simulink model "fusionAlg"  (R2018b)
settings: Solver=FixedStepDiscrete  StartTime=0.0  StopTime=inf  FixedStep=0.01  RelTol=1e-3
PostLoadFcn:
  | if any(exist('dsrtsu_mdlpostloadfcn', 'file') ~= 0), dsrtsu_mdlpostloadfcn('Execute', bdroot); end
model workspace (MAT data in the model file):
  handle : class17 (value not decoded)
(part 4 of 24)

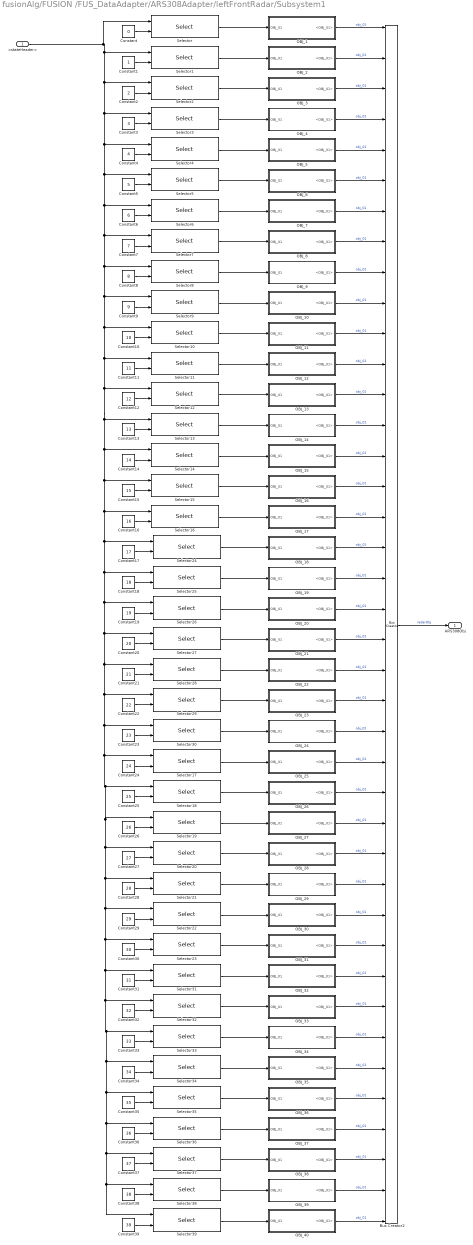
== system fusionAlg/FUSION /FUS_DataAdapter/ARS308Adapter/leftFrontRadar/Subsystem1 ==
  <stateHeader> : Inport
  Bus Creator2 : BusCreator  Inputs=40  OutDataTypeStr=Bus: FUS_RADOBJ_LIST_ST  NonVirtualBus=on
      settings: InheritFromInputs=off
  Constant : Constant  Value=0  OutDataTypeStr=uint8
  Constant1 : Constant  OutDataTypeStr=uint8
  Constant10 : Constant  Value=10  OutDataTypeStr=uint8
  Constant11 : Constant  Value=11  OutDataTypeStr=uint8
  Constant12 : Constant  Value=12  OutDataTypeStr=uint8
  Constant13 : Constant  Value=13  OutDataTypeStr=uint8
  Constant14 : Constant  Value=14  OutDataTypeStr=uint8
  Constant15 : Constant  Value=15  OutDataTypeStr=uint8
  Constant16 : Constant  Value=16  OutDataTypeStr=uint8
  Constant17 : Constant  Value=17  OutDataTypeStr=uint8
  Constant18 : Constant  Value=18  OutDataTypeStr=uint8
  Constant19 : Constant  Value=19  OutDataTypeStr=uint8
  Constant2 : Constant  Value=2  OutDataTypeStr=uint8
  Constant20 : Constant  Value=20  OutDataTypeStr=uint8
  Constant21 : Constant  Value=21  OutDataTypeStr=uint8
  Constant22 : Constant  Value=22  OutDataTypeStr=uint8
  Constant23 : Constant  Value=23  OutDataTypeStr=uint8
  Constant24 : Constant  Value=24  OutDataTypeStr=uint8
  Constant25 : Constant  Value=25  OutDataTypeStr=uint8
  Constant26 : Constant  Value=26  OutDataTypeStr=uint8
  Constant27 : Constant  Value=27  OutDataTypeStr=uint8
  Constant28 : Constant  Value=28  OutDataTypeStr=uint8
  Constant29 : Constant  Value=29  OutDataTypeStr=uint8
  Constant3 : Constant  Value=3  OutDataTypeStr=uint8
  Constant30 : Constant  Value=30  OutDataTypeStr=uint8
  Constant31 : Constant  Value=31  OutDataTypeStr=uint8
  Constant32 : Constant  Value=32  OutDataTypeStr=uint8
  Constant33 : Constant  Value=33  OutDataTypeStr=uint8
  Constant34 : Constant  Value=34  OutDataTypeStr=uint8
  Constant35 : Constant  Value=35  OutDataTypeStr=uint8
  Constant36 : Constant  Value=36  OutDataTypeStr=uint8
  Constant37 : Constant  Value=37  OutDataTypeStr=uint8
  Constant38 : Constant  Value=38  OutDataTypeStr=uint8
  Constant39 : Constant  Value=39  OutDataTypeStr=uint8
  Constant4 : Constant  Value=4  OutDataTypeStr=uint8
  Constant5 : Constant  Value=5  OutDataTypeStr=uint8
  Constant6 : Constant  Value=6  OutDataTypeStr=uint8
  Constant7 : Constant  Value=7  OutDataTypeStr=uint8
  Constant8 : Constant  Value=8  OutDataTypeStr=uint8
  Constant9 : Constant  Value=9  OutDataTypeStr=uint8
  OBJ_1 : Subsystem
  OBJ_10 : Subsystem
  OBJ_11 : Subsystem
  OBJ_12 : Subsystem
  OBJ_13 : Subsystem
  OBJ_14 : Subsystem
  OBJ_15 : Subsystem
  OBJ_16 : Subsystem
  OBJ_17 : Subsystem
  OBJ_18 : Subsystem
  OBJ_19 : Subsystem
  OBJ_2 : Subsystem
  OBJ_20 : Subsystem
  OBJ_21 : Subsystem
  OBJ_22 : Subsystem
  OBJ_23 : Subsystem
  OBJ_24 : Subsystem
  OBJ_25 : Subsystem
  OBJ_26 : Subsystem
  OBJ_27 : Subsystem
  OBJ_28 : Subsystem
  OBJ_29 : Subsystem
  OBJ_3 : Subsystem
  OBJ_30 : Subsystem
  OBJ_31 : Subsystem
  OBJ_32 : Subsystem
  OBJ_33 : Subsystem
  OBJ_34 : Subsystem
  OBJ_35 : Subsystem
  OBJ_36 : Subsystem
  OBJ_37 : Subsystem
  OBJ_38 : Subsystem
  OBJ_39 : Subsystem
  OBJ_4 : Subsystem
  OBJ_40 : Subsystem
  OBJ_5 : Subsystem
  OBJ_6 : Subsystem
  OBJ_7 : Subsystem
  OBJ_8 : Subsystem
  OBJ_9 : Subsystem
  Selector{,1..39} (40 alike) : Selector  IndexMode=Zero-based  InputPortWidth=40  IndexOptions=Index vector (port)  Indices=[1 3]  OutputSizes=1
  ARS308Obj : Outport
  wires:
  Bus Creator2/1 -> ARS308Obj/1  "radarObj"
  Constant/1 -> Selector/2
  Constant11/1 -> Selector11/2
  Constant2/1 -> Selector2/2
  Constant5/1 -> Selector5/2
  Constant26/1 -> Selector19/2
  Constant3/1 -> Selector3/2
  Constant34/1 -> Selector34/2
  Constant22/1 -> Selector29/2
  Constant9/1 -> Selector9/2
  Constant38/1 -> Selector38/2
  Constant14/1 -> Selector14/2
  Constant23/1 -> Selector30/2
  Constant1/1 -> Selector1/2
  Constant6/1 -> Selector6/2
  Constant4/1 -> Selector4/2
  Constant8/1 -> Selector8/2
  <stateHeader>/1 -> Selector/1, Selector9/1, Selector39/1, Selector38/1, Selector37/1, Selector36/1, Selector35/1, Selector34/1, Selector33/1, Selector32/1, Selector31/1, Selector23/1, Selector22/1, Selector21/1, Selector20/1, Selector19/1, Selector18/1, Selector17/1, Selector30/1, Selector29/1, Selector28/1, Selector27/1, Selector26/1, Selector25/1, Selector24/1, Selector16/1, Selector15/1, Selector14/1, Selector13/1, Selector12/1, Selector11/1, Selector10/1, Selector8/1, Selector7/1, Selector6/1, Selector5/1, Selector4/1, Selector3/1, Selector2/1, Selector1/1
  Selector/1 -> OBJ_1/1(OBJ_01)
  Constant17/1 -> Selector24/2
  Constant12/1 -> Selector12/2
  Constant20/1 -> Selector27/2
  Constant39/1 -> Selector39/2
  Constant37/1 -> Selector37/2
  Constant36/1 -> Selector36/2
  Constant15/1 -> Selector15/2
  Constant10/1 -> Selector10/2
  Constant18/1 -> Selector25/2
  Constant19/1 -> Selector26/2
  Constant16/1 -> Selector16/2
  Constant25/1 -> Selector18/2
  Constant28/1 -> Selector21/2
  Constant31/1 -> Selector31/2
  Constant29/1 -> Selector22/2
  Constant13/1 -> Selector13/2
  Constant33/1 -> Selector33/2
  Constant32/1 -> Selector32/2
  Constant24/1 -> Selector17/2
  Constant21/1 -> Selector28/2
  Constant30/1 -> Selector23/2
  Constant27/1 -> Selector20/2
  Constant7/1 -> Selector7/2
  Constant35/1 -> Selector35/2
  OBJ_1/1(<OBJ_01>) -> Bus Creator2/1  "obj_01"
  Selector1/1 -> OBJ_2/1(OBJ_01)
  OBJ_2/1(<OBJ_01>) -> Bus Creator2/2  "obj_01"
  Selector2/1 -> OBJ_3/1(OBJ_01)
  Selector3/1 -> OBJ_4/1(OBJ_01)
  OBJ_4/1(<OBJ_01>) -> Bus Creator2/4  "obj_01"
  OBJ_3/1(<OBJ_01>) -> Bus Creator2/3  "obj_01"
  Selector7/1 -> OBJ_8/1(OBJ_01)
  Selector4/1 -> OBJ_5/1(OBJ_01)
  Selector5/1 -> OBJ_6/1(OBJ_01)
  Selector6/1 -> OBJ_7/1(OBJ_01)
  OBJ_7/1(<OBJ_01>) -> Bus Creator2/7  "obj_01"
  OBJ_6/1(<OBJ_01>) -> Bus Creator2/6  "obj_01"
  OBJ_5/1(<OBJ_01>) -> Bus Creator2/5  "obj_01"
  OBJ_8/1(<OBJ_01>) -> Bus Creator2/8  "obj_01"
  Selector8/1 -> OBJ_9/1(OBJ_01)
  Selector10/1 -> OBJ_11/1(OBJ_01)
  OBJ_10/1(<OBJ_01>) -> Bus Creator2/10  "obj_01"
  OBJ_11/1(<OBJ_01>) -> Bus Creator2/11  "obj_01"
  Selector12/1 -> OBJ_13/1(OBJ_01)
  Selector9/1 -> OBJ_10/1(OBJ_01)
  Selector11/1 -> OBJ_12/1(OBJ_01)
  OBJ_9/1(<OBJ_01>) -> Bus Creator2/9  "obj_01"
  OBJ_13/1(<OBJ_01>) -> Bus Creator2/13  "obj_01"
  OBJ_12/1(<OBJ_01>) -> Bus Creator2/12  "obj_01"
  Selector13/1 -> OBJ_14/1(OBJ_01)
  OBJ_17/1(<OBJ_01>) -> Bus Creator2/17  "obj_01"
  OBJ_14/1(<OBJ_01>) -> Bus Creator2/14  "obj_01"
  OBJ_16/1(<OBJ_01>) -> Bus Creator2/16  "obj_01"
  OBJ_15/1(<OBJ_01>) -> Bus Creator2/15  "obj_01"
  Selector15/1 -> OBJ_16/1(OBJ_01)
  Selector14/1 -> OBJ_15/1(OBJ_01)
  Selector16/1 -> OBJ_17/1(OBJ_01)
  Selector27/1 -> OBJ_21/1(OBJ_01)
  Selector26/1 -> OBJ_20/1(OBJ_01)
  OBJ_18/1(<OBJ_01>) -> Bus Creator2/18  "obj_01"
  OBJ_20/1(<OBJ_01>) -> Bus Creator2/20  "obj_01"
  OBJ_19/1(<OBJ_01>) -> Bus Creator2/19  "obj_01"
  Selector24/1 -> OBJ_18/1(OBJ_01)
  OBJ_21/1(<OBJ_01>) -> Bus Creator2/21  "obj_01"
  Selector25/1 -> OBJ_19/1(OBJ_01)
  Selector28/1 -> OBJ_22/1(OBJ_01)
  OBJ_22/1(<OBJ_01>) -> Bus Creator2/22  "obj_01"
  Selector17/1 -> OBJ_25/1(OBJ_01)
  Selector30/1 -> OBJ_24/1(OBJ_01)
  Selector29/1 -> OBJ_23/1(OBJ_01)
  OBJ_24/1(<OBJ_01>) -> Bus Creator2/24  "obj_01"
  OBJ_23/1(<OBJ_01>) -> Bus Creator2/23  "obj_01"
  OBJ_25/1(<OBJ_01>) -> Bus Creator2/25  "obj_01"
  OBJ_26/1(<OBJ_01>) -> Bus Creator2/26  "obj_01"
  Selector18/1 -> OBJ_26/1(OBJ_01)
  Selector22/1 -> OBJ_30/1(OBJ_01)
  OBJ_27/1(<OBJ_01>) -> Bus Creator2/27  "obj_01"
  Selector21/1 -> OBJ_29/1(OBJ_01)
  OBJ_30/1(<OBJ_01>) -> Bus Creator2/30  "obj_01"
  Selector20/1 -> OBJ_28/1(OBJ_01)
  Selector19/1 -> OBJ_27/1(OBJ_01)
  Selector23/1 -> OBJ_31/1(OBJ_01)
  OBJ_31/1(<OBJ_01>) -> Bus Creator2/31  "obj_01"
  OBJ_29/1(<OBJ_01>) -> Bus Creator2/29  "obj_01"
  OBJ_28/1(<OBJ_01>) -> Bus Creator2/28  "obj_01"
  OBJ_33/1(<OBJ_01>) -> Bus Creator2/33  "obj_01"
  OBJ_34/1(<OBJ_01>) -> Bus Creator2/34  "obj_01"
  Selector34/1 -> OBJ_35/1(OBJ_01)
  Selector33/1 -> OBJ_34/1(OBJ_01)
  Selector32/1 -> OBJ_33/1(OBJ_01)
  OBJ_32/1(<OBJ_01>) -> Bus Creator2/32  "obj_01"
  OBJ_36/1(<OBJ_01>) -> Bus Creator2/36  "obj_01"
  Selector35/1 -> OBJ_36/1(OBJ_01)
  OBJ_35/1(<OBJ_01>) -> Bus Creator2/35  "obj_01"
  Selector31/1 -> OBJ_32/1(OBJ_01)
  Selector39/1 -> OBJ_40/1(OBJ_01)
  OBJ_37/1(<OBJ_01>) -> Bus Creator2/37  "obj_01"
  Selector36/1 -> OBJ_37/1(OBJ_01)
  Selector38/1 -> OBJ_39/1(OBJ_01)
  OBJ_38/1(<OBJ_01>) -> Bus Creator2/38  "obj_01"
  OBJ_40/1(<OBJ_01>) -> Bus Creator2/40  "obj_01"
  Selector37/1 -> OBJ_38/1(OBJ_01)
  OBJ_39/1(<OBJ_01>) -> Bus Creator2/39  "obj_01"

== system fusionAlg/FUSION /FUS_DataAdapter/ARS308Adapter/leftFrontRadar/Subsystem40 ==
  <MeasCounter> : Inport
  Bus Creator1 : BusCreator  Inputs=12  OutDataTypeStr=Bus: FUS_RADAR_STATE_ST  NonVirtualBus=on
      settings: InheritFromInputs=off
  Bus Creator2 : BusCreator  Inputs=2  OutDataTypeStr=Bus: FUS_UINT8_RESERVED_ST  NonVirtualBus=on
      settings: InheritFromInputs=off
  Constant{,1,5..11} (9 alike) : Constant  Value=0  OutDataTypeStr=uint8
  Constant2 : Constant  Value=0  OutDataTypeStr=single
  Constant3 : Constant  Value=0  OutDataTypeStr=single
  Constant4 : Constant  Value=0  OutDataTypeStr=uint16
  Data Type Conversion : DataTypeConversion  OutDataTypeStr=uint8
  <STATUS> : Outport
  wires:
  Constant/1 -> Bus Creator2/1
  <MeasCounter>/1 -> Data Type Conversion/1
  Constant1/1 -> Bus Creator2/2
  Bus Creator2/1 -> Bus Creator1/12
  Bus Creator1/1 -> <STATUS>/1
  Constant2/1 -> Bus Creator1/1  "hostYaw"
  Constant3/1 -> Bus Creator1/2  "hostSpeed"
  Constant4/1 -> Bus Creator1/3  "timestamp"
  Constant5/1 -> Bus Creator1/4  "HWError"
  Constant6/1 -> Bus Creator1/5  "BlkProg"
  Constant7/1 -> Bus Creator1/6  "MisAlign"
  Constant8/1 -> Bus Creator1/7  "GUFail"
  Constant9/1 -> Bus Creator1/8  "measEnabled"
  Constant10/1 -> Bus Creator1/10  "latency"
  Constant11/1 -> Bus Creator1/11  "msgCheckSum"
  Data Type Conversion/1 -> Bus Creator1/9

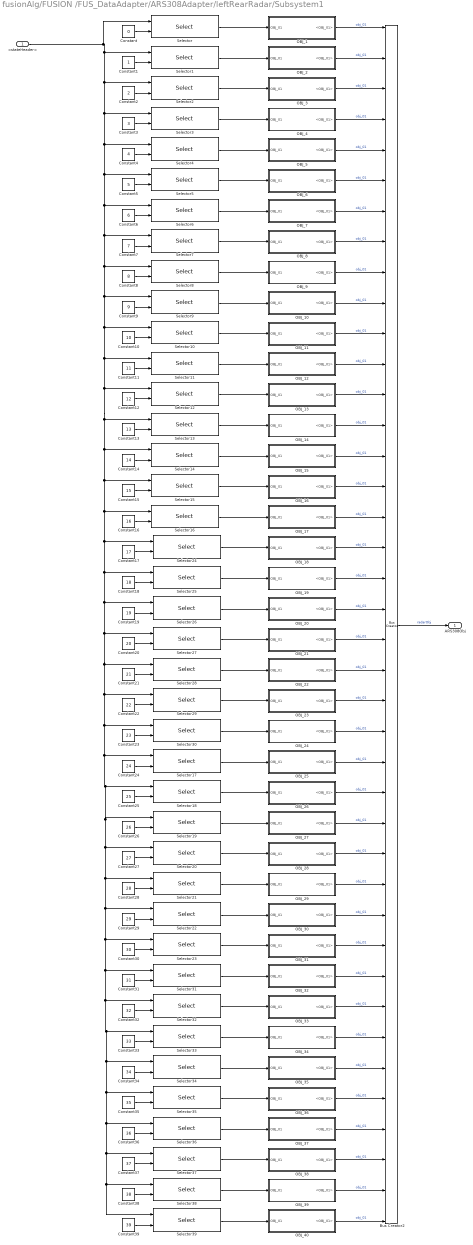
== system fusionAlg/FUSION /FUS_DataAdapter/ARS308Adapter/leftRearRadar/Subsystem1 ==
  <stateHeader> : Inport
  Bus Creator2 : BusCreator  Inputs=40  OutDataTypeStr=Bus: FUS_RADOBJ_LIST_ST  NonVirtualBus=on
      settings: InheritFromInputs=off
  Constant : Constant  Value=0  OutDataTypeStr=uint8
  Constant1 : Constant  OutDataTypeStr=uint8
  Constant10 : Constant  Value=10  OutDataTypeStr=uint8
  Constant11 : Constant  Value=11  OutDataTypeStr=uint8
  Constant12 : Constant  Value=12  OutDataTypeStr=uint8
  Constant13 : Constant  Value=13  OutDataTypeStr=uint8
  Constant14 : Constant  Value=14  OutDataTypeStr=uint8
  Constant15 : Constant  Value=15  OutDataTypeStr=uint8
  Constant16 : Constant  Value=16  OutDataTypeStr=uint8
  Constant17 : Constant  Value=17  OutDataTypeStr=uint8
  Constant18 : Constant  Value=18  OutDataTypeStr=uint8
  Constant19 : Constant  Value=19  OutDataTypeStr=uint8
  Constant2 : Constant  Value=2  OutDataTypeStr=uint8
  Constant20 : Constant  Value=20  OutDataTypeStr=uint8
  Constant21 : Constant  Value=21  OutDataTypeStr=uint8
  Constant22 : Constant  Value=22  OutDataTypeStr=uint8
  Constant23 : Constant  Value=23  OutDataTypeStr=uint8
  Constant24 : Constant  Value=24  OutDataTypeStr=uint8
  Constant25 : Constant  Value=25  OutDataTypeStr=uint8
  Constant26 : Constant  Value=26  OutDataTypeStr=uint8
  Constant27 : Constant  Value=27  OutDataTypeStr=uint8
  Constant28 : Constant  Value=28  OutDataTypeStr=uint8
  Constant29 : Constant  Value=29  OutDataTypeStr=uint8
  Constant3 : Constant  Value=3  OutDataTypeStr=uint8
  Constant30 : Constant  Value=30  OutDataTypeStr=uint8
  Constant31 : Constant  Value=31  OutDataTypeStr=uint8
  Constant32 : Constant  Value=32  OutDataTypeStr=uint8
  Constant33 : Constant  Value=33  OutDataTypeStr=uint8
  Constant34 : Constant  Value=34  OutDataTypeStr=uint8
  Constant35 : Constant  Value=35  OutDataTypeStr=uint8
  Constant36 : Constant  Value=36  OutDataTypeStr=uint8
  Constant37 : Constant  Value=37  OutDataTypeStr=uint8
  Constant38 : Constant  Value=38  OutDataTypeStr=uint8
  Constant39 : Constant  Value=39  OutDataTypeStr=uint8
  Constant4 : Constant  Value=4  OutDataTypeStr=uint8
  Constant5 : Constant  Value=5  OutDataTypeStr=uint8
  Constant6 : Constant  Value=6  OutDataTypeStr=uint8
  Constant7 : Constant  Value=7  OutDataTypeStr=uint8
  Constant8 : Constant  Value=8  OutDataTypeStr=uint8
  Constant9 : Constant  Value=9  OutDataTypeStr=uint8
  OBJ_1 : Subsystem
  OBJ_10 : Subsystem
  OBJ_11 : Subsystem
  OBJ_12 : Subsystem
  OBJ_13 : Subsystem
  OBJ_14 : Subsystem
  OBJ_15 : Subsystem
  OBJ_16 : Subsystem
  OBJ_17 : Subsystem
  OBJ_18 : Subsystem
  OBJ_19 : Subsystem
  OBJ_2 : Subsystem
  OBJ_20 : Subsystem
  OBJ_21 : Subsystem
  OBJ_22 : Subsystem
  OBJ_23 : Subsystem
  OBJ_24 : Subsystem
  OBJ_25 : Subsystem
  OBJ_26 : Subsystem
  OBJ_27 : Subsystem
  OBJ_28 : Subsystem
  OBJ_29 : Subsystem
  OBJ_3 : Subsystem
  OBJ_30 : Subsystem
  OBJ_31 : Subsystem
  OBJ_32 : Subsystem
  OBJ_33 : Subsystem
  OBJ_34 : Subsystem
  OBJ_35 : Subsystem
  OBJ_36 : Subsystem
  OBJ_37 : Subsystem
  OBJ_38 : Subsystem
  OBJ_39 : Subsystem
  OBJ_4 : Subsystem
  OBJ_40 : Subsystem
  OBJ_5 : Subsystem
  OBJ_6 : Subsystem
  OBJ_7 : Subsystem
  OBJ_8 : Subsystem
  OBJ_9 : Subsystem
  Selector{,1..39} (40 alike) : Selector  IndexMode=Zero-based  InputPortWidth=40  IndexOptions=Index vector (port)  Indices=[1 3]  OutputSizes=1
  ARS308Obj : Outport
  wires:
  Bus Creator2/1 -> ARS308Obj/1  "radarObj"
  Constant/1 -> Selector/2
  Constant11/1 -> Selector11/2
  Constant2/1 -> Selector2/2
  Constant5/1 -> Selector5/2
  Constant26/1 -> Selector19/2
  Constant3/1 -> Selector3/2
  Constant34/1 -> Selector34/2
  Constant22/1 -> Selector29/2
  Constant9/1 -> Selector9/2
  Constant38/1 -> Selector38/2
  Constant14/1 -> Selector14/2
  Constant23/1 -> Selector30/2
  Constant1/1 -> Selector1/2
  Constant6/1 -> Selector6/2
  Constant4/1 -> Selector4/2
  Constant8/1 -> Selector8/2
  <stateHeader>/1 -> Selector/1, Selector9/1, Selector39/1, Selector38/1, Selector37/1, Selector36/1, Selector35/1, Selector34/1, Selector33/1, Selector32/1, Selector31/1, Selector23/1, Selector22/1, Selector21/1, Selector20/1, Selector19/1, Selector18/1, Selector17/1, Selector30/1, Selector29/1, Selector28/1, Selector27/1, Selector26/1, Selector25/1, Selector24/1, Selector16/1, Selector15/1, Selector14/1, Selector13/1, Selector12/1, Selector11/1, Selector10/1, Selector8/1, Selector7/1, Selector6/1, Selector5/1, Selector4/1, Selector3/1, Selector2/1, Selector1/1
  Selector/1 -> OBJ_1/1(OBJ_01)
  Constant17/1 -> Selector24/2
  Constant12/1 -> Selector12/2
  Constant20/1 -> Selector27/2
  Constant39/1 -> Selector39/2
  Constant37/1 -> Selector37/2
  Constant36/1 -> Selector36/2
  Constant15/1 -> Selector15/2
  Constant10/1 -> Selector10/2
  Constant18/1 -> Selector25/2
  Constant19/1 -> Selector26/2
  Constant16/1 -> Selector16/2
  Constant25/1 -> Selector18/2
  Constant28/1 -> Selector21/2
  Constant31/1 -> Selector31/2
  Constant29/1 -> Selector22/2
  Constant13/1 -> Selector13/2
  Constant33/1 -> Selector33/2
  Constant32/1 -> Selector32/2
  Constant24/1 -> Selector17/2
  Constant21/1 -> Selector28/2
  Constant30/1 -> Selector23/2
  Constant27/1 -> Selector20/2
  Constant7/1 -> Selector7/2
  Constant35/1 -> Selector35/2
  OBJ_1/1(<OBJ_01>) -> Bus Creator2/1  "obj_01"
  Selector1/1 -> OBJ_2/1(OBJ_01)
  OBJ_2/1(<OBJ_01>) -> Bus Creator2/2  "obj_01"
  Selector2/1 -> OBJ_3/1(OBJ_01)
  Selector3/1 -> OBJ_4/1(OBJ_01)
  OBJ_4/1(<OBJ_01>) -> Bus Creator2/4  "obj_01"
  OBJ_3/1(<OBJ_01>) -> Bus Creator2/3  "obj_01"
  Selector7/1 -> OBJ_8/1(OBJ_01)
  Selector4/1 -> OBJ_5/1(OBJ_01)
  Selector5/1 -> OBJ_6/1(OBJ_01)
  Selector6/1 -> OBJ_7/1(OBJ_01)
  OBJ_7/1(<OBJ_01>) -> Bus Creator2/7  "obj_01"
  OBJ_6/1(<OBJ_01>) -> Bus Creator2/6  "obj_01"
  OBJ_5/1(<OBJ_01>) -> Bus Creator2/5  "obj_01"
  OBJ_8/1(<OBJ_01>) -> Bus Creator2/8  "obj_01"
  Selector8/1 -> OBJ_9/1(OBJ_01)
  Selector10/1 -> OBJ_11/1(OBJ_01)
  OBJ_10/1(<OBJ_01>) -> Bus Creator2/10  "obj_01"
  OBJ_11/1(<OBJ_01>) -> Bus Creator2/11  "obj_01"
  Selector12/1 -> OBJ_13/1(OBJ_01)
  Selector9/1 -> OBJ_10/1(OBJ_01)
  Selector11/1 -> OBJ_12/1(OBJ_01)
  OBJ_9/1(<OBJ_01>) -> Bus Creator2/9  "obj_01"
  OBJ_13/1(<OBJ_01>) -> Bus Creator2/13  "obj_01"
  OBJ_12/1(<OBJ_01>) -> Bus Creator2/12  "obj_01"
  Selector13/1 -> OBJ_14/1(OBJ_01)
  OBJ_17/1(<OBJ_01>) -> Bus Creator2/17  "obj_01"
  OBJ_14/1(<OBJ_01>) -> Bus Creator2/14  "obj_01"
  OBJ_16/1(<OBJ_01>) -> Bus Creator2/16  "obj_01"
  OBJ_15/1(<OBJ_01>) -> Bus Creator2/15  "obj_01"
  Selector15/1 -> OBJ_16/1(OBJ_01)
  Selector14/1 -> OBJ_15/1(OBJ_01)
  Selector16/1 -> OBJ_17/1(OBJ_01)
  Selector27/1 -> OBJ_21/1(OBJ_01)
  Selector26/1 -> OBJ_20/1(OBJ_01)
  OBJ_18/1(<OBJ_01>) -> Bus Creator2/18  "obj_01"
  OBJ_20/1(<OBJ_01>) -> Bus Creator2/20  "obj_01"
  OBJ_19/1(<OBJ_01>) -> Bus Creator2/19  "obj_01"
  Selector24/1 -> OBJ_18/1(OBJ_01)
  OBJ_21/1(<OBJ_01>) -> Bus Creator2/21  "obj_01"
  Selector25/1 -> OBJ_19/1(OBJ_01)
  Selector28/1 -> OBJ_22/1(OBJ_01)
  OBJ_22/1(<OBJ_01>) -> Bus Creator2/22  "obj_01"
  Selector17/1 -> OBJ_25/1(OBJ_01)
  Selector30/1 -> OBJ_24/1(OBJ_01)
  Selector29/1 -> OBJ_23/1(OBJ_01)
  OBJ_24/1(<OBJ_01>) -> Bus Creator2/24  "obj_01"
  OBJ_23/1(<OBJ_01>) -> Bus Creator2/23  "obj_01"
  OBJ_25/1(<OBJ_01>) -> Bus Creator2/25  "obj_01"
  OBJ_26/1(<OBJ_01>) -> Bus Creator2/26  "obj_01"
  Selector18/1 -> OBJ_26/1(OBJ_01)
  Selector22/1 -> OBJ_30/1(OBJ_01)
  OBJ_27/1(<OBJ_01>) -> Bus Creator2/27  "obj_01"
  Selector21/1 -> OBJ_29/1(OBJ_01)
  OBJ_30/1(<OBJ_01>) -> Bus Creator2/30  "obj_01"
  Selector20/1 -> OBJ_28/1(OBJ_01)
  Selector19/1 -> OBJ_27/1(OBJ_01)
  Selector23/1 -> OBJ_31/1(OBJ_01)
  OBJ_31/1(<OBJ_01>) -> Bus Creator2/31  "obj_01"
  OBJ_29/1(<OBJ_01>) -> Bus Creator2/29  "obj_01"
  OBJ_28/1(<OBJ_01>) -> Bus Creator2/28  "obj_01"
  OBJ_33/1(<OBJ_01>) -> Bus Creator2/33  "obj_01"
  OBJ_34/1(<OBJ_01>) -> Bus Creator2/34  "obj_01"
  Selector34/1 -> OBJ_35/1(OBJ_01)
  Selector33/1 -> OBJ_34/1(OBJ_01)
  Selector32/1 -> OBJ_33/1(OBJ_01)
  OBJ_32/1(<OBJ_01>) -> Bus Creator2/32  "obj_01"
  OBJ_36/1(<OBJ_01>) -> Bus Creator2/36  "obj_01"
  Selector35/1 -> OBJ_36/1(OBJ_01)
  OBJ_35/1(<OBJ_01>) -> Bus Creator2/35  "obj_01"
  Selector31/1 -> OBJ_32/1(OBJ_01)
  Selector39/1 -> OBJ_40/1(OBJ_01)
  OBJ_37/1(<OBJ_01>) -> Bus Creator2/37  "obj_01"
  Selector36/1 -> OBJ_37/1(OBJ_01)
  Selector38/1 -> OBJ_39/1(OBJ_01)
  OBJ_38/1(<OBJ_01>) -> Bus Creator2/38  "obj_01"
  OBJ_40/1(<OBJ_01>) -> Bus Creator2/40  "obj_01"
  Selector37/1 -> OBJ_38/1(OBJ_01)
  OBJ_39/1(<OBJ_01>) -> Bus Creator2/39  "obj_01"

== system fusionAlg/FUSION /FUS_DataAdapter/ARS308Adapter/leftRearRadar/Subsystem40 ==
  <MeasCounter> : Inport
  Bus Creator1 : BusCreator  Inputs=12  OutDataTypeStr=Bus: FUS_RADAR_STATE_ST  NonVirtualBus=on
      settings: InheritFromInputs=off
  Bus Creator2 : BusCreator  Inputs=2  OutDataTypeStr=Bus: FUS_UINT8_RESERVED_ST  NonVirtualBus=on
      settings: InheritFromInputs=off
  Constant{,1,5..11} (9 alike) : Constant  Value=0  OutDataTypeStr=uint8
  Constant2 : Constant  Value=0  OutDataTypeStr=single
  Constant3 : Constant  Value=0  OutDataTypeStr=single
  Constant4 : Constant  Value=0  OutDataTypeStr=uint16
  Data Type Conversion : DataTypeConversion  OutDataTypeStr=uint8
  <STATUS> : Outport
  wires:
  Constant/1 -> Bus Creator2/1
  <MeasCounter>/1 -> Data Type Conversion/1
  Constant1/1 -> Bus Creator2/2
  Bus Creator2/1 -> Bus Creator1/12
  Bus Creator1/1 -> <STATUS>/1
  Constant2/1 -> Bus Creator1/1  "hostYaw"
  Constant3/1 -> Bus Creator1/2  "hostSpeed"
  Constant4/1 -> Bus Creator1/3  "timestamp"
  Constant5/1 -> Bus Creator1/4  "HWError"
  Constant6/1 -> Bus Creator1/5  "BlkProg"
  Constant7/1 -> Bus Creator1/6  "MisAlign"
  Constant8/1 -> Bus Creator1/7  "GUFail"
  Constant9/1 -> Bus Creator1/8  "measEnabled"
  Constant10/1 -> Bus Creator1/10  "latency"
  Constant11/1 -> Bus Creator1/11  "msgCheckSum"
  Data Type Conversion/1 -> Bus Creator1/9

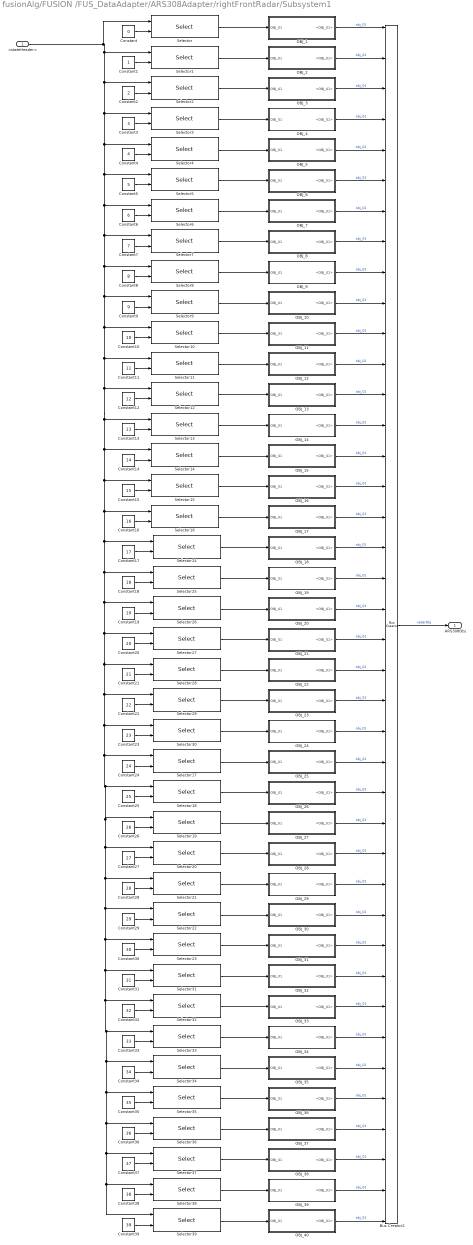
== system fusionAlg/FUSION /FUS_DataAdapter/ARS308Adapter/rightFrontRadar/Subsystem1 ==
  <stateHeader> : Inport
  Bus Creator2 : BusCreator  Inputs=40  OutDataTypeStr=Bus: FUS_RADOBJ_LIST_ST  NonVirtualBus=on
      settings: InheritFromInputs=off
  Constant : Constant  Value=0  OutDataTypeStr=uint8
  Constant1 : Constant  OutDataTypeStr=uint8
  Constant10 : Constant  Value=10  OutDataTypeStr=uint8
  Constant11 : Constant  Value=11  OutDataTypeStr=uint8
  Constant12 : Constant  Value=12  OutDataTypeStr=uint8
  Constant13 : Constant  Value=13  OutDataTypeStr=uint8
  Constant14 : Constant  Value=14  OutDataTypeStr=uint8
  Constant15 : Constant  Value=15  OutDataTypeStr=uint8
  Constant16 : Constant  Value=16  OutDataTypeStr=uint8
  Constant17 : Constant  Value=17  OutDataTypeStr=uint8
  Constant18 : Constant  Value=18  OutDataTypeStr=uint8
  Constant19 : Constant  Value=19  OutDataTypeStr=uint8
  Constant2 : Constant  Value=2  OutDataTypeStr=uint8
  Constant20 : Constant  Value=20  OutDataTypeStr=uint8
  Constant21 : Constant  Value=21  OutDataTypeStr=uint8
  Constant22 : Constant  Value=22  OutDataTypeStr=uint8
  Constant23 : Constant  Value=23  OutDataTypeStr=uint8
  Constant24 : Constant  Value=24  OutDataTypeStr=uint8
  Constant25 : Constant  Value=25  OutDataTypeStr=uint8
  Constant26 : Constant  Value=26  OutDataTypeStr=uint8
  Constant27 : Constant  Value=27  OutDataTypeStr=uint8
  Constant28 : Constant  Value=28  OutDataTypeStr=uint8
  Constant29 : Constant  Value=29  OutDataTypeStr=uint8
  Constant3 : Constant  Value=3  OutDataTypeStr=uint8
  Constant30 : Constant  Value=30  OutDataTypeStr=uint8
  Constant31 : Constant  Value=31  OutDataTypeStr=uint8
  Constant32 : Constant  Value=32  OutDataTypeStr=uint8
  Constant33 : Constant  Value=33  OutDataTypeStr=uint8
  Constant34 : Constant  Value=34  OutDataTypeStr=uint8
  Constant35 : Constant  Value=35  OutDataTypeStr=uint8
  Constant36 : Constant  Value=36  OutDataTypeStr=uint8
  Constant37 : Constant  Value=37  OutDataTypeStr=uint8
  Constant38 : Constant  Value=38  OutDataTypeStr=uint8
  Constant39 : Constant  Value=39  OutDataTypeStr=uint8
  Constant4 : Constant  Value=4  OutDataTypeStr=uint8
  Constant5 : Constant  Value=5  OutDataTypeStr=uint8
  Constant6 : Constant  Value=6  OutDataTypeStr=uint8
  Constant7 : Constant  Value=7  OutDataTypeStr=uint8
  Constant8 : Constant  Value=8  OutDataTypeStr=uint8
  Constant9 : Constant  Value=9  OutDataTypeStr=uint8
  OBJ_1 : Subsystem
  OBJ_10 : Subsystem
  OBJ_11 : Subsystem
  OBJ_12 : Subsystem
  OBJ_13 : Subsystem
  OBJ_14 : Subsystem
  OBJ_15 : Subsystem
  OBJ_16 : Subsystem
  OBJ_17 : Subsystem
  OBJ_18 : Subsystem
  OBJ_19 : Subsystem
  OBJ_2 : Subsystem
  OBJ_20 : Subsystem
  OBJ_21 : Subsystem
  OBJ_22 : Subsystem
  OBJ_23 : Subsystem
  OBJ_24 : Subsystem
  OBJ_25 : Subsystem
  OBJ_26 : Subsystem
  OBJ_27 : Subsystem
  OBJ_28 : Subsystem
  OBJ_29 : Subsystem
  OBJ_3 : Subsystem
  OBJ_30 : Subsystem
  OBJ_31 : Subsystem
  OBJ_32 : Subsystem
  OBJ_33 : Subsystem
  OBJ_34 : Subsystem
  OBJ_35 : Subsystem
  OBJ_36 : Subsystem
  OBJ_37 : Subsystem
  OBJ_38 : Subsystem
  OBJ_39 : Subsystem
  OBJ_4 : Subsystem
  OBJ_40 : Subsystem
  OBJ_5 : Subsystem
  OBJ_6 : Subsystem
  OBJ_7 : Subsystem
  OBJ_8 : Subsystem
  OBJ_9 : Subsystem
  Selector{,1..39} (40 alike) : Selector  IndexMode=Zero-based  InputPortWidth=40  IndexOptions=Index vector (port)  Indices=[1 3]  OutputSizes=1
  ARS308Obj : Outport
  wires:
  Bus Creator2/1 -> ARS308Obj/1  "radarObj"
  Constant/1 -> Selector/2
  Constant11/1 -> Selector11/2
  Constant2/1 -> Selector2/2
  Constant5/1 -> Selector5/2
  Constant26/1 -> Selector19/2
  Constant3/1 -> Selector3/2
  Constant34/1 -> Selector34/2
  Constant22/1 -> Selector29/2
  Constant9/1 -> Selector9/2
  Constant38/1 -> Selector38/2
  Constant14/1 -> Selector14/2
  Constant23/1 -> Selector30/2
  Constant1/1 -> Selector1/2
  Constant6/1 -> Selector6/2
  Constant4/1 -> Selector4/2
  Constant8/1 -> Selector8/2
  <stateHeader>/1 -> Selector/1, Selector9/1, Selector39/1, Selector38/1, Selector37/1, Selector36/1, Selector35/1, Selector34/1, Selector33/1, Selector32/1, Selector31/1, Selector23/1, Selector22/1, Selector21/1, Selector20/1, Selector19/1, Selector18/1, Selector17/1, Selector30/1, Selector29/1, Selector28/1, Selector27/1, Selector26/1, Selector25/1, Selector24/1, Selector16/1, Selector15/1, Selector14/1, Selector13/1, Selector12/1, Selector11/1, Selector10/1, Selector8/1, Selector7/1, Selector6/1, Selector5/1, Selector4/1, Selector3/1, Selector2/1, Selector1/1
  Selector/1 -> OBJ_1/1(OBJ_01)
  Constant17/1 -> Selector24/2
  Constant12/1 -> Selector12/2
  Constant20/1 -> Selector27/2
  Constant39/1 -> Selector39/2
  Constant37/1 -> Selector37/2
  Constant36/1 -> Selector36/2
  Constant15/1 -> Selector15/2
  Constant10/1 -> Selector10/2
  Constant18/1 -> Selector25/2
  Constant19/1 -> Selector26/2
  Constant16/1 -> Selector16/2
  Constant25/1 -> Selector18/2
  Constant28/1 -> Selector21/2
  Constant31/1 -> Selector31/2
  Constant29/1 -> Selector22/2
  Constant13/1 -> Selector13/2
  Constant33/1 -> Selector33/2
  Constant32/1 -> Selector32/2
  Constant24/1 -> Selector17/2
  Constant21/1 -> Selector28/2
  Constant30/1 -> Selector23/2
  Constant27/1 -> Selector20/2
  Constant7/1 -> Selector7/2
  Constant35/1 -> Selector35/2
  OBJ_1/1(<OBJ_01>) -> Bus Creator2/1  "obj_01"
  Selector1/1 -> OBJ_2/1(OBJ_01)
  OBJ_2/1(<OBJ_01>) -> Bus Creator2/2  "obj_01"
  Selector2/1 -> OBJ_3/1(OBJ_01)
  Selector3/1 -> OBJ_4/1(OBJ_01)
  OBJ_4/1(<OBJ_01>) -> Bus Creator2/4  "obj_01"
  OBJ_3/1(<OBJ_01>) -> Bus Creator2/3  "obj_01"
  Selector7/1 -> OBJ_8/1(OBJ_01)
  Selector4/1 -> OBJ_5/1(OBJ_01)
  Selector5/1 -> OBJ_6/1(OBJ_01)
  Selector6/1 -> OBJ_7/1(OBJ_01)
  OBJ_7/1(<OBJ_01>) -> Bus Creator2/7  "obj_01"
  OBJ_6/1(<OBJ_01>) -> Bus Creator2/6  "obj_01"
  OBJ_5/1(<OBJ_01>) -> Bus Creator2/5  "obj_01"
  OBJ_8/1(<OBJ_01>) -> Bus Creator2/8  "obj_01"
  Selector8/1 -> OBJ_9/1(OBJ_01)
  Selector10/1 -> OBJ_11/1(OBJ_01)
  OBJ_10/1(<OBJ_01>) -> Bus Creator2/10  "obj_01"
  OBJ_11/1(<OBJ_01>) -> Bus Creator2/11  "obj_01"
  Selector12/1 -> OBJ_13/1(OBJ_01)
  Selector9/1 -> OBJ_10/1(OBJ_01)
  Selector11/1 -> OBJ_12/1(OBJ_01)
  OBJ_9/1(<OBJ_01>) -> Bus Creator2/9  "obj_01"
  OBJ_13/1(<OBJ_01>) -> Bus Creator2/13  "obj_01"
  OBJ_12/1(<OBJ_01>) -> Bus Creator2/12  "obj_01"
  Selector13/1 -> OBJ_14/1(OBJ_01)
  OBJ_17/1(<OBJ_01>) -> Bus Creator2/17  "obj_01"
  OBJ_14/1(<OBJ_01>) -> Bus Creator2/14  "obj_01"
  OBJ_16/1(<OBJ_01>) -> Bus Creator2/16  "obj_01"
  OBJ_15/1(<OBJ_01>) -> Bus Creator2/15  "obj_01"
  Selector15/1 -> OBJ_16/1(OBJ_01)
  Selector14/1 -> OBJ_15/1(OBJ_01)
  Selector16/1 -> OBJ_17/1(OBJ_01)
  Selector27/1 -> OBJ_21/1(OBJ_01)
  Selector26/1 -> OBJ_20/1(OBJ_01)
  OBJ_18/1(<OBJ_01>) -> Bus Creator2/18  "obj_01"
  OBJ_20/1(<OBJ_01>) -> Bus Creator2/20  "obj_01"
  OBJ_19/1(<OBJ_01>) -> Bus Creator2/19  "obj_01"
  Selector24/1 -> OBJ_18/1(OBJ_01)
  OBJ_21/1(<OBJ_01>) -> Bus Creator2/21  "obj_01"
  Selector25/1 -> OBJ_19/1(OBJ_01)
  Selector28/1 -> OBJ_22/1(OBJ_01)
  OBJ_22/1(<OBJ_01>) -> Bus Creator2/22  "obj_01"
  Selector17/1 -> OBJ_25/1(OBJ_01)
  Selector30/1 -> OBJ_24/1(OBJ_01)
  Selector29/1 -> OBJ_23/1(OBJ_01)
  OBJ_24/1(<OBJ_01>) -> Bus Creator2/24  "obj_01"
  OBJ_23/1(<OBJ_01>) -> Bus Creator2/23  "obj_01"
  OBJ_25/1(<OBJ_01>) -> Bus Creator2/25  "obj_01"
  OBJ_26/1(<OBJ_01>) -> Bus Creator2/26  "obj_01"
  Selector18/1 -> OBJ_26/1(OBJ_01)
  Selector22/1 -> OBJ_30/1(OBJ_01)
  OBJ_27/1(<OBJ_01>) -> Bus Creator2/27  "obj_01"
  Selector21/1 -> OBJ_29/1(OBJ_01)
  OBJ_30/1(<OBJ_01>) -> Bus Creator2/30  "obj_01"
  Selector20/1 -> OBJ_28/1(OBJ_01)
  Selector19/1 -> OBJ_27/1(OBJ_01)
  Selector23/1 -> OBJ_31/1(OBJ_01)
  OBJ_31/1(<OBJ_01>) -> Bus Creator2/31  "obj_01"
  OBJ_29/1(<OBJ_01>) -> Bus Creator2/29  "obj_01"
  OBJ_28/1(<OBJ_01>) -> Bus Creator2/28  "obj_01"
  OBJ_33/1(<OBJ_01>) -> Bus Creator2/33  "obj_01"
  OBJ_34/1(<OBJ_01>) -> Bus Creator2/34  "obj_01"
  Selector34/1 -> OBJ_35/1(OBJ_01)
  Selector33/1 -> OBJ_34/1(OBJ_01)
  Selector32/1 -> OBJ_33/1(OBJ_01)
  OBJ_32/1(<OBJ_01>) -> Bus Creator2/32  "obj_01"
  OBJ_36/1(<OBJ_01>) -> Bus Creator2/36  "obj_01"
  Selector35/1 -> OBJ_36/1(OBJ_01)
  OBJ_35/1(<OBJ_01>) -> Bus Creator2/35  "obj_01"
  Selector31/1 -> OBJ_32/1(OBJ_01)
  Selector39/1 -> OBJ_40/1(OBJ_01)
  OBJ_37/1(<OBJ_01>) -> Bus Creator2/37  "obj_01"
  Selector36/1 -> OBJ_37/1(OBJ_01)
  Selector38/1 -> OBJ_39/1(OBJ_01)
  OBJ_38/1(<OBJ_01>) -> Bus Creator2/38  "obj_01"
  OBJ_40/1(<OBJ_01>) -> Bus Creator2/40  "obj_01"
  Selector37/1 -> OBJ_38/1(OBJ_01)
  OBJ_39/1(<OBJ_01>) -> Bus Creator2/39  "obj_01"

== system fusionAlg/FUSION /FUS_DataAdapter/ARS308Adapter/rightFrontRadar/Subsystem40 ==
  <MeasCounter> : Inport
  Bus Creator1 : BusCreator  Inputs=12  OutDataTypeStr=Bus: FUS_RADAR_STATE_ST  NonVirtualBus=on
      settings: InheritFromInputs=off
  Bus Creator2 : BusCreator  Inputs=2  OutDataTypeStr=Bus: FUS_UINT8_RESERVED_ST  NonVirtualBus=on
      settings: InheritFromInputs=off
  Constant{,1,5..11} (9 alike) : Constant  Value=0  OutDataTypeStr=uint8
  Constant2 : Constant  Value=0  OutDataTypeStr=single
  Constant3 : Constant  Value=0  OutDataTypeStr=single
  Constant4 : Constant  Value=0  OutDataTypeStr=uint16
  Data Type Conversion : DataTypeConversion  OutDataTypeStr=uint8
  <STATUS> : Outport
  wires:
  Constant/1 -> Bus Creator2/1
  <MeasCounter>/1 -> Data Type Conversion/1
  Constant1/1 -> Bus Creator2/2
  Bus Creator2/1 -> Bus Creator1/12
  Bus Creator1/1 -> <STATUS>/1
  Constant2/1 -> Bus Creator1/1  "hostYaw"
  Constant3/1 -> Bus Creator1/2  "hostSpeed"
  Constant4/1 -> Bus Creator1/3  "timestamp"
  Constant5/1 -> Bus Creator1/4  "HWError"
  Constant6/1 -> Bus Creator1/5  "BlkProg"
  Constant7/1 -> Bus Creator1/6  "MisAlign"
  Constant8/1 -> Bus Creator1/7  "GUFail"
  Constant9/1 -> Bus Creator1/8  "measEnabled"
  Constant10/1 -> Bus Creator1/10  "latency"
  Constant11/1 -> Bus Creator1/11  "msgCheckSum"
  Data Type Conversion/1 -> Bus Creator1/9

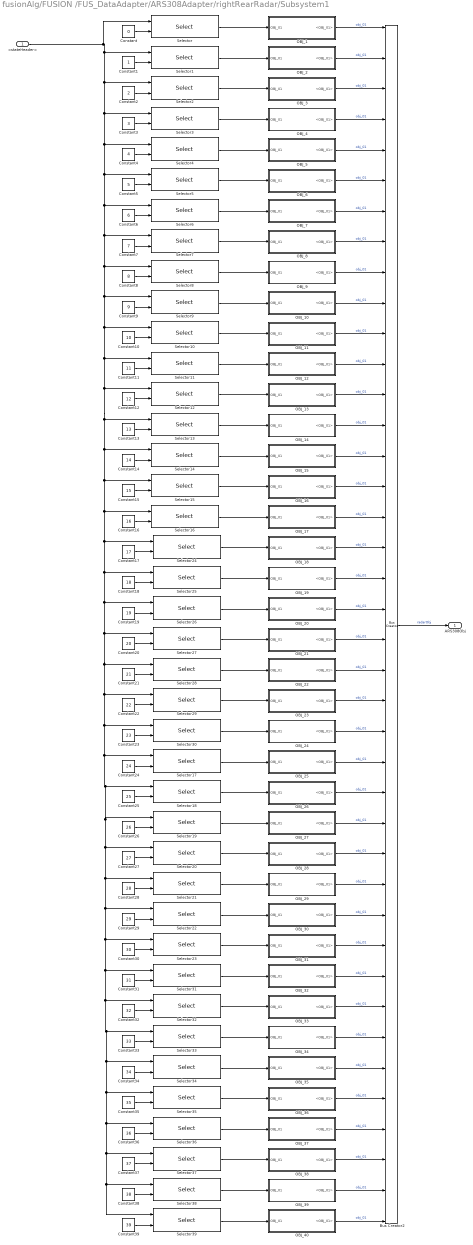
== system fusionAlg/FUSION /FUS_DataAdapter/ARS308Adapter/rightRearRadar/Subsystem1 ==
  <stateHeader> : Inport
  Bus Creator2 : BusCreator  Inputs=40  OutDataTypeStr=Bus: FUS_RADOBJ_LIST_ST  NonVirtualBus=on
      settings: InheritFromInputs=off
  Constant : Constant  Value=0  OutDataTypeStr=uint8
  Constant1 : Constant  OutDataTypeStr=uint8
  Constant10 : Constant  Value=10  OutDataTypeStr=uint8
  Constant11 : Constant  Value=11  OutDataTypeStr=uint8
  Constant12 : Constant  Value=12  OutDataTypeStr=uint8
  Constant13 : Constant  Value=13  OutDataTypeStr=uint8
  Constant14 : Constant  Value=14  OutDataTypeStr=uint8
  Constant15 : Constant  Value=15  OutDataTypeStr=uint8
  Constant16 : Constant  Value=16  OutDataTypeStr=uint8
  Constant17 : Constant  Value=17  OutDataTypeStr=uint8
  Constant18 : Constant  Value=18  OutDataTypeStr=uint8
  Constant19 : Constant  Value=19  OutDataTypeStr=uint8
  Constant2 : Constant  Value=2  OutDataTypeStr=uint8
  Constant20 : Constant  Value=20  OutDataTypeStr=uint8
  Constant21 : Constant  Value=21  OutDataTypeStr=uint8
  Constant22 : Constant  Value=22  OutDataTypeStr=uint8
  Constant23 : Constant  Value=23  OutDataTypeStr=uint8
  Constant24 : Constant  Value=24  OutDataTypeStr=uint8
  Constant25 : Constant  Value=25  OutDataTypeStr=uint8
  Constant26 : Constant  Value=26  OutDataTypeStr=uint8
  Constant27 : Constant  Value=27  OutDataTypeStr=uint8
  Constant28 : Constant  Value=28  OutDataTypeStr=uint8
  Constant29 : Constant  Value=29  OutDataTypeStr=uint8
  Constant3 : Constant  Value=3  OutDataTypeStr=uint8
  Constant30 : Constant  Value=30  OutDataTypeStr=uint8
  Constant31 : Constant  Value=31  OutDataTypeStr=uint8
  Constant32 : Constant  Value=32  OutDataTypeStr=uint8
  Constant33 : Constant  Value=33  OutDataTypeStr=uint8
  Constant34 : Constant  Value=34  OutDataTypeStr=uint8
  Constant35 : Constant  Value=35  OutDataTypeStr=uint8
  Constant36 : Constant  Value=36  OutDataTypeStr=uint8
  Constant37 : Constant  Value=37  OutDataTypeStr=uint8
  Constant38 : Constant  Value=38  OutDataTypeStr=uint8
  Constant39 : Constant  Value=39  OutDataTypeStr=uint8
  Constant4 : Constant  Value=4  OutDataTypeStr=uint8
  Constant5 : Constant  Value=5  OutDataTypeStr=uint8
  Constant6 : Constant  Value=6  OutDataTypeStr=uint8
  Constant7 : Constant  Value=7  OutDataTypeStr=uint8
  Constant8 : Constant  Value=8  OutDataTypeStr=uint8
  Constant9 : Constant  Value=9  OutDataTypeStr=uint8
  OBJ_1 : Subsystem
  OBJ_10 : Subsystem
  OBJ_11 : Subsystem
  OBJ_12 : Subsystem
  OBJ_13 : Subsystem
  OBJ_14 : Subsystem
  OBJ_15 : Subsystem
  OBJ_16 : Subsystem
  OBJ_17 : Subsystem
  OBJ_18 : Subsystem
  OBJ_19 : Subsystem
  OBJ_2 : Subsystem
  OBJ_20 : Subsystem
  OBJ_21 : Subsystem
  OBJ_22 : Subsystem
  OBJ_23 : Subsystem
  OBJ_24 : Subsystem
  OBJ_25 : Subsystem
  OBJ_26 : Subsystem
  OBJ_27 : Subsystem
  OBJ_28 : Subsystem
  OBJ_29 : Subsystem
  OBJ_3 : Subsystem
  OBJ_30 : Subsystem
  OBJ_31 : Subsystem
  OBJ_32 : Subsystem
  OBJ_33 : Subsystem
  OBJ_34 : Subsystem
  OBJ_35 : Subsystem
  OBJ_36 : Subsystem
  OBJ_37 : Subsystem
  OBJ_38 : Subsystem
  OBJ_39 : Subsystem
  OBJ_4 : Subsystem
  OBJ_40 : Subsystem
  OBJ_5 : Subsystem
  OBJ_6 : Subsystem
  OBJ_7 : Subsystem
  OBJ_8 : Subsystem
  OBJ_9 : Subsystem
  Selector{,1..39} (40 alike) : Selector  IndexMode=Zero-based  InputPortWidth=40  IndexOptions=Index vector (port)  Indices=[1 3]  OutputSizes=1
  ARS308Obj : Outport
  wires:
  Bus Creator2/1 -> ARS308Obj/1  "radarObj"
  Constant/1 -> Selector/2
  Constant11/1 -> Selector11/2
  Constant2/1 -> Selector2/2
  Constant5/1 -> Selector5/2
  Constant26/1 -> Selector19/2
  Constant3/1 -> Selector3/2
  Constant34/1 -> Selector34/2
  Constant22/1 -> Selector29/2
  Constant9/1 -> Selector9/2
  Constant38/1 -> Selector38/2
  Constant14/1 -> Selector14/2
  Constant23/1 -> Selector30/2
  Constant1/1 -> Selector1/2
  Constant6/1 -> Selector6/2
  Constant4/1 -> Selector4/2
  Constant8/1 -> Selector8/2
  <stateHeader>/1 -> Selector/1, Selector9/1, Selector39/1, Selector38/1, Selector37/1, Selector36/1, Selector35/1, Selector34/1, Selector33/1, Selector32/1, Selector31/1, Selector23/1, Selector22/1, Selector21/1, Selector20/1, Selector19/1, Selector18/1, Selector17/1, Selector30/1, Selector29/1, Selector28/1, Selector27/1, Selector26/1, Selector25/1, Selector24/1, Selector16/1, Selector15/1, Selector14/1, Selector13/1, Selector12/1, Selector11/1, Selector10/1, Selector8/1, Selector7/1, Selector6/1, Selector5/1, Selector4/1, Selector3/1, Selector2/1, Selector1/1
  Selector/1 -> OBJ_1/1(OBJ_01)
  Constant17/1 -> Selector24/2
  Constant12/1 -> Selector12/2
  Constant20/1 -> Selector27/2
  Constant39/1 -> Selector39/2
  Constant37/1 -> Selector37/2
  Constant36/1 -> Selector36/2
  Constant15/1 -> Selector15/2
  Constant10/1 -> Selector10/2
  Constant18/1 -> Selector25/2
  Constant19/1 -> Selector26/2
  Constant16/1 -> Selector16/2
  Constant25/1 -> Selector18/2
  Constant28/1 -> Selector21/2
  Constant31/1 -> Selector31/2
  Constant29/1 -> Selector22/2
  Constant13/1 -> Selector13/2
  Constant33/1 -> Selector33/2
  Constant32/1 -> Selector32/2
  Constant24/1 -> Selector17/2
  Constant21/1 -> Selector28/2
  Constant30/1 -> Selector23/2
  Constant27/1 -> Selector20/2
  Constant7/1 -> Selector7/2
  Constant35/1 -> Selector35/2
  OBJ_1/1(<OBJ_01>) -> Bus Creator2/1  "obj_01"
  Selector1/1 -> OBJ_2/1(OBJ_01)
  OBJ_2/1(<OBJ_01>) -> Bus Creator2/2  "obj_01"
  Selector2/1 -> OBJ_3/1(OBJ_01)
  Selector3/1 -> OBJ_4/1(OBJ_01)
  OBJ_4/1(<OBJ_01>) -> Bus Creator2/4  "obj_01"
  OBJ_3/1(<OBJ_01>) -> Bus Creator2/3  "obj_01"
  Selector7/1 -> OBJ_8/1(OBJ_01)
  Selector4/1 -> OBJ_5/1(OBJ_01)
  Selector5/1 -> OBJ_6/1(OBJ_01)
  Selector6/1 -> OBJ_7/1(OBJ_01)
  OBJ_7/1(<OBJ_01>) -> Bus Creator2/7  "obj_01"
  OBJ_6/1(<OBJ_01>) -> Bus Creator2/6  "obj_01"
  OBJ_5/1(<OBJ_01>) -> Bus Creator2/5  "obj_01"
  OBJ_8/1(<OBJ_01>) -> Bus Creator2/8  "obj_01"
  Selector8/1 -> OBJ_9/1(OBJ_01)
  Selector10/1 -> OBJ_11/1(OBJ_01)
  OBJ_10/1(<OBJ_01>) -> Bus Creator2/10  "obj_01"
  OBJ_11/1(<OBJ_01>) -> Bus Creator2/11  "obj_01"
  Selector12/1 -> OBJ_13/1(OBJ_01)
  Selector9/1 -> OBJ_10/1(OBJ_01)
  Selector11/1 -> OBJ_12/1(OBJ_01)
  OBJ_9/1(<OBJ_01>) -> Bus Creator2/9  "obj_01"
  OBJ_13/1(<OBJ_01>) -> Bus Creator2/13  "obj_01"
  OBJ_12/1(<OBJ_01>) -> Bus Creator2/12  "obj_01"
  Selector13/1 -> OBJ_14/1(OBJ_01)
  OBJ_17/1(<OBJ_01>) -> Bus Creator2/17  "obj_01"
  OBJ_14/1(<OBJ_01>) -> Bus Creator2/14  "obj_01"
  OBJ_16/1(<OBJ_01>) -> Bus Creator2/16  "obj_01"
  OBJ_15/1(<OBJ_01>) -> Bus Creator2/15  "obj_01"
  Selector15/1 -> OBJ_16/1(OBJ_01)
  Selector14/1 -> OBJ_15/1(OBJ_01)
  Selector16/1 -> OBJ_17/1(OBJ_01)
  Selector27/1 -> OBJ_21/1(OBJ_01)
  Selector26/1 -> OBJ_20/1(OBJ_01)
  OBJ_18/1(<OBJ_01>) -> Bus Creator2/18  "obj_01"
  OBJ_20/1(<OBJ_01>) -> Bus Creator2/20  "obj_01"
  OBJ_19/1(<OBJ_01>) -> Bus Creator2/19  "obj_01"
  Selector24/1 -> OBJ_18/1(OBJ_01)
  OBJ_21/1(<OBJ_01>) -> Bus Creator2/21  "obj_01"
  Selector25/1 -> OBJ_19/1(OBJ_01)
  Selector28/1 -> OBJ_22/1(OBJ_01)
  OBJ_22/1(<OBJ_01>) -> Bus Creator2/22  "obj_01"
  Selector17/1 -> OBJ_25/1(OBJ_01)
  Selector30/1 -> OBJ_24/1(OBJ_01)
  Selector29/1 -> OBJ_23/1(OBJ_01)
  OBJ_24/1(<OBJ_01>) -> Bus Creator2/24  "obj_01"
  OBJ_23/1(<OBJ_01>) -> Bus Creator2/23  "obj_01"
  OBJ_25/1(<OBJ_01>) -> Bus Creator2/25  "obj_01"
  OBJ_26/1(<OBJ_01>) -> Bus Creator2/26  "obj_01"
  Selector18/1 -> OBJ_26/1(OBJ_01)
  Selector22/1 -> OBJ_30/1(OBJ_01)
  OBJ_27/1(<OBJ_01>) -> Bus Creator2/27  "obj_01"
  Selector21/1 -> OBJ_29/1(OBJ_01)
  OBJ_30/1(<OBJ_01>) -> Bus Creator2/30  "obj_01"
  Selector20/1 -> OBJ_28/1(OBJ_01)
  Selector19/1 -> OBJ_27/1(OBJ_01)
  Selector23/1 -> OBJ_31/1(OBJ_01)
  OBJ_31/1(<OBJ_01>) -> Bus Creator2/31  "obj_01"
  OBJ_29/1(<OBJ_01>) -> Bus Creator2/29  "obj_01"
  OBJ_28/1(<OBJ_01>) -> Bus Creator2/28  "obj_01"
  OBJ_33/1(<OBJ_01>) -> Bus Creator2/33  "obj_01"
  OBJ_34/1(<OBJ_01>) -> Bus Creator2/34  "obj_01"
  Selector34/1 -> OBJ_35/1(OBJ_01)
  Selector33/1 -> OBJ_34/1(OBJ_01)
  Selector32/1 -> OBJ_33/1(OBJ_01)
  OBJ_32/1(<OBJ_01>) -> Bus Creator2/32  "obj_01"
  OBJ_36/1(<OBJ_01>) -> Bus Creator2/36  "obj_01"
  Selector35/1 -> OBJ_36/1(OBJ_01)
  OBJ_35/1(<OBJ_01>) -> Bus Creator2/35  "obj_01"
  Selector31/1 -> OBJ_32/1(OBJ_01)
  Selector39/1 -> OBJ_40/1(OBJ_01)
  OBJ_37/1(<OBJ_01>) -> Bus Creator2/37  "obj_01"
  Selector36/1 -> OBJ_37/1(OBJ_01)
  Selector38/1 -> OBJ_39/1(OBJ_01)
  OBJ_38/1(<OBJ_01>) -> Bus Creator2/38  "obj_01"
  OBJ_40/1(<OBJ_01>) -> Bus Creator2/40  "obj_01"
  Selector37/1 -> OBJ_38/1(OBJ_01)
  OBJ_39/1(<OBJ_01>) -> Bus Creator2/39  "obj_01"

== system fusionAlg/FUSION /FUS_DataAdapter/ARS308Adapter/rightRearRadar/Subsystem40 ==
  <MeasCounter> : Inport
  Bus Creator1 : BusCreator  Inputs=12  OutDataTypeStr=Bus: FUS_RADAR_STATE_ST  NonVirtualBus=on
      settings: InheritFromInputs=off
  Bus Creator2 : BusCreator  Inputs=2  OutDataTypeStr=Bus: FUS_UINT8_RESERVED_ST  NonVirtualBus=on
      settings: InheritFromInputs=off
  Constant{,1,5..11} (9 alike) : Constant  Value=0  OutDataTypeStr=uint8
  Constant2 : Constant  Value=0  OutDataTypeStr=single
  Constant3 : Constant  Value=0  OutDataTypeStr=single
  Constant4 : Constant  Value=0  OutDataTypeStr=uint16
  Data Type Conversion : DataTypeConversion  OutDataTypeStr=uint8
  <STATUS> : Outport
  wires:
  Constant/1 -> Bus Creator2/1
  <MeasCounter>/1 -> Data Type Conversion/1
  Constant1/1 -> Bus Creator2/2
  Bus Creator2/1 -> Bus Creator1/12
  Bus Creator1/1 -> <STATUS>/1
  Constant2/1 -> Bus Creator1/1  "hostYaw"
  Constant3/1 -> Bus Creator1/2  "hostSpeed"
  Constant4/1 -> Bus Creator1/3  "timestamp"
  Constant5/1 -> Bus Creator1/4  "HWError"
  Constant6/1 -> Bus Creator1/5  "BlkProg"
  Constant7/1 -> Bus Creator1/6  "MisAlign"
  Constant8/1 -> Bus Creator1/7  "GUFail"
  Constant9/1 -> Bus Creator1/8  "measEnabled"
  Constant10/1 -> Bus Creator1/10  "latency"
  Constant11/1 -> Bus Creator1/11  "msgCheckSum"
  Data Type Conversion/1 -> Bus Creator1/9

== system fusionAlg/FUSION /FUS_DataAdapter/VisionAdapter/LaneAdapter/Lane_AdjaA ==
  EyeQ4_AdjaA : Inport
  Bus Creator1 : BusCreator  Inputs=17  OutDataTypeStr=Bus: FUS_EYEQ4_LANE_ADJA_ST  NonVirtualBus=on
      settings: InheritFromInputs=off
  Bus Selector : BusSelector  OutputSignals=LA_Line_C0,LA_Line_C1,LA_Line_C2,LA_Line_C3,LA_Line_Role,LA_Lane_Track_ID,LA_Age,LA_Color,LA_Color_Conf,LA_Marker_Width,LA_Marker_Width_STD,LA_View_Range_Start,LA_View_Range_End,LA_Exist_Probability,LA_Lanemark_Type,LA_Lanemark_Type_Conf,LA_DLM_Type
  Data Type Conversion{,1..7} (8 alike) : DataTypeConversion  OutDataTypeStr=uint32
  Lane_AdjaA_st : Outport  OutDataTypeStr=Bus: FUS_EYEQ4_LANE_ADJA_ST
  wires:
  Bus Creator1/1 -> Lane_AdjaA_st/1
  EyeQ4_AdjaA/1 -> Bus Selector/1
  Bus Selector/1 -> Bus Creator1/1  "<LA_Line_C0>"
  Bus Selector/2 -> Bus Creator1/2  "<LA_Line_C1>"
  Bus Selector/3 -> Bus Creator1/3  "<LA_Line_C2>"
  Bus Selector/4 -> Bus Creator1/4  "<LA_Line_C3>"
  Bus Selector/5 -> Data Type Conversion/1  "<LA_Line_Role>"
  Bus Selector/6 -> Data Type Conversion1/1  "<LA_Lane_Track_ID>"
  Bus Selector/7 -> Data Type Conversion2/1  "<LA_Age>"
  Bus Selector/8 -> Data Type Conversion3/1  "<LA_Color>"
  Bus Selector/9 -> Data Type Conversion4/1  "<LA_Color_Conf>"
  Bus Selector/10 -> Bus Creator1/10  "<LA_Marker_Width>"
  Bus Selector/11 -> Bus Creator1/11  "<LA_Marker_Width_STD>"
  Bus Selector/12 -> Bus Creator1/12  "<LA_View_Range_Start>"
  Bus Selector/13 -> Bus Creator1/13  "<LA_View_Range_End>"
  Bus Selector/14 -> Bus Creator1/14  "<LA_Exist_Probability>"
  Bus Selector/15 -> Data Type Conversion5/1  "<LA_Lanemark_Type>"
  Bus Selector/16 -> Data Type Conversion6/1  "<LA_Lanemark_Type_Conf>"
  Data Type Conversion/1 -> Bus Creator1/5  "LA_Line_Role"
  Data Type Conversion1/1 -> Bus Creator1/6  "LA_Lane_Track_ID"
  Data Type Conversion2/1 -> Bus Creator1/7  "LA_Age"
  Data Type Conversion3/1 -> Bus Creator1/8  "LA_Color"
  Data Type Conversion4/1 -> Bus Creator1/9  "LA_Color_Conf"
  Data Type Conversion5/1 -> Bus Creator1/15  "LA_LaneMark_Type"
  Data Type Conversion6/1 -> Bus Creator1/16  "LA_LaneMark_Type_Conf"
  Bus Selector/17 -> Data Type Conversion7/1  "<LA_DLM_Type>"
  Data Type Conversion7/1 -> Bus Creator1/17  "LA_Type"

== system fusionAlg/FUSION /FUS_DataAdapter/VisionAdapter/LaneAdapter/Lane_AdjaB ==
  EyeQ4_AdjaB : Inport
  Bus Creator1 : BusCreator  Inputs=17  OutDataTypeStr=Bus: FUS_EYEQ4_LANE_ADJA_ST  NonVirtualBus=on
      settings: InheritFromInputs=off
  Bus Selector : BusSelector  OutputSignals=LA_Line_C0,LA_Line_C1,LA_Line_C2,LA_Line_C3,LA_Line_Role,LA_Lane_Track_ID,LA_Age,LA_Color,LA_Color_Conf,LA_Marker_Width,LA_Marker_Width_STD,LA_View_Range_Start,LA_View_Range_End,LA_Exist_Probability,LA_Lanemark_Type,LA_Lanemark_Type_Conf,LA_DLM_Type
  Data Type Conversion{,1..7} (8 alike) : DataTypeConversion  OutDataTypeStr=uint32
  Lane_AdjaB_st : Outport  OutDataTypeStr=Bus: FUS_EYEQ4_LANE_ADJA_ST
  wires:
  Bus Creator1/1 -> Lane_AdjaB_st/1
  EyeQ4_AdjaB/1 -> Bus Selector/1
  Bus Selector/1 -> Bus Creator1/1  "<LA_Line_C0>"
  Bus Selector/2 -> Bus Creator1/2  "<LA_Line_C1>"
  Bus Selector/3 -> Bus Creator1/3  "<LA_Line_C2>"
  Bus Selector/4 -> Bus Creator1/4  "<LA_Line_C3>"
  Bus Selector/5 -> Data Type Conversion/1  "<LA_Line_Role>"
  Bus Selector/6 -> Data Type Conversion1/1  "<LA_Lane_Track_ID>"
  Bus Selector/7 -> Data Type Conversion2/1  "<LA_Age>"
  Bus Selector/8 -> Data Type Conversion3/1  "<LA_Color>"
  Bus Selector/9 -> Data Type Conversion4/1  "<LA_Color_Conf>"
  Bus Selector/10 -> Bus Creator1/10  "<LA_Marker_Width>"
  Bus Selector/11 -> Bus Creator1/11  "<LA_Marker_Width_STD>"
  Bus Selector/12 -> Bus Creator1/12  "<LA_View_Range_Start>"
  Bus Selector/13 -> Bus Creator1/13  "<LA_View_Range_End>"
  Bus Selector/14 -> Bus Creator1/14  "<LA_Exist_Probability>"
  Bus Selector/15 -> Data Type Conversion5/1  "<LA_Lanemark_Type>"
  Bus Selector/16 -> Data Type Conversion6/1  "<LA_Lanemark_Type_Conf>"
  Data Type Conversion/1 -> Bus Creator1/5  "LA_Line_Role"
  Data Type Conversion1/1 -> Bus Creator1/6  "LA_Lane_Track_ID"
  Data Type Conversion2/1 -> Bus Creator1/7  "LA_Age"
  Data Type Conversion3/1 -> Bus Creator1/8  "LA_Color"
  Data Type Conversion4/1 -> Bus Creator1/9  "LA_Color_Conf"
  Data Type Conversion5/1 -> Bus Creator1/15  "LA_LaneMark_Type"
  Data Type Conversion6/1 -> Bus Creator1/16  "LA_LaneMark_Type_Conf"
  Bus Selector/17 -> Data Type Conversion7/1  "<LA_DLM_Type>"
  Data Type Conversion7/1 -> Bus Creator1/17  "LA_Type"

== system fusionAlg/FUSION /FUS_DataAdapter/VisionAdapter/LaneAdapter/Lane_AdjaC ==
  EyeQ4_AdjaC : Inport
  Bus Creator1 : BusCreator  Inputs=17  OutDataTypeStr=Bus: FUS_EYEQ4_LANE_ADJA_ST  NonVirtualBus=on
      settings: InheritFromInputs=off
  Bus Selector : BusSelector  OutputSignals=LA_Line_C0,LA_Line_C1,LA_Line_C2,LA_Line_C3,LA_Line_Role,LA_Lane_Track_ID,LA_Age,LA_Color,LA_Color_Conf,LA_Marker_Width,LA_Marker_Width_STD,LA_View_Range_Start,LA_View_Range_End,LA_Exist_Probability,LA_Lanemark_Type,LA_Lanemark_Type_Conf,LA_DLM_Type
  Data Type Conversion{,1..7} (8 alike) : DataTypeConversion  OutDataTypeStr=uint32
  Lane_AdjaC_st : Outport  OutDataTypeStr=Bus: FUS_EYEQ4_LANE_ADJA_ST
  wires:
  Bus Creator1/1 -> Lane_AdjaC_st/1
  EyeQ4_AdjaC/1 -> Bus Selector/1
  Bus Selector/1 -> Bus Creator1/1  "<LA_Line_C0>"
  Bus Selector/2 -> Bus Creator1/2  "<LA_Line_C1>"
  Bus Selector/3 -> Bus Creator1/3  "<LA_Line_C2>"
  Bus Selector/4 -> Bus Creator1/4  "<LA_Line_C3>"
  Bus Selector/5 -> Data Type Conversion/1  "<LA_Line_Role>"
  Bus Selector/6 -> Data Type Conversion1/1  "<LA_Lane_Track_ID>"
  Bus Selector/7 -> Data Type Conversion2/1  "<LA_Age>"
  Bus Selector/8 -> Data Type Conversion3/1  "<LA_Color>"
  Bus Selector/9 -> Data Type Conversion4/1  "<LA_Color_Conf>"
  Bus Selector/10 -> Bus Creator1/10  "<LA_Marker_Width>"
  Bus Selector/11 -> Bus Creator1/11  "<LA_Marker_Width_STD>"
  Bus Selector/12 -> Bus Creator1/12  "<LA_View_Range_Start>"
  Bus Selector/13 -> Bus Creator1/13  "<LA_View_Range_End>"
  Bus Selector/14 -> Bus Creator1/14  "<LA_Exist_Probability>"
  Bus Selector/15 -> Data Type Conversion5/1  "<LA_Lanemark_Type>"
  Bus Selector/16 -> Data Type Conversion6/1  "<LA_Lanemark_Type_Conf>"
  Data Type Conversion/1 -> Bus Creator1/5  "LA_Line_Role"
  Data Type Conversion1/1 -> Bus Creator1/6  "LA_Lane_Track_ID"
  Data Type Conversion2/1 -> Bus Creator1/7  "LA_Age"
  Data Type Conversion3/1 -> Bus Creator1/8  "LA_Color"
  Data Type Conversion4/1 -> Bus Creator1/9  "LA_Color_Conf"
  Data Type Conversion5/1 -> Bus Creator1/15  "LA_LaneMark_Type"
  Data Type Conversion6/1 -> Bus Creator1/16  "LA_LaneMark_Type_Conf"
  Bus Selector/17 -> Data Type Conversion7/1  "<LA_DLM_Type>"
  Data Type Conversion7/1 -> Bus Creator1/17  "LA_Type"

== system fusionAlg/FUSION /FUS_DataAdapter/VisionAdapter/LaneAdapter/Lane_AdjaD ==
  EyeQ4_AdjaD : Inport
  Bus Creator1 : BusCreator  Inputs=17  OutDataTypeStr=Bus: FUS_EYEQ4_LANE_ADJA_ST  NonVirtualBus=on
      settings: InheritFromInputs=off
  Bus Selector : BusSelector  OutputSignals=LA_Line_C0,LA_Line_C1,LA_Line_C2,LA_Line_C3,LA_Line_Role,LA_Lane_Track_ID,LA_Age,LA_Color,LA_Color_Conf,LA_Marker_Width,LA_Marker_Width_STD,LA_View_Range_Start,LA_View_Range_End,LA_Exist_Probability,LA_Lanemark_Type,LA_Lanemark_Type_Conf,LA_DLM_Type
  Data Type Conversion{,1..7} (8 alike) : DataTypeConversion  OutDataTypeStr=uint32
  Lane_AdjaD_st : Outport  OutDataTypeStr=Bus: FUS_EYEQ4_LANE_ADJA_ST
  wires:
  Bus Creator1/1 -> Lane_AdjaD_st/1
  EyeQ4_AdjaD/1 -> Bus Selector/1
  Bus Selector/1 -> Bus Creator1/1  "<LA_Line_C0>"
  Bus Selector/2 -> Bus Creator1/2  "<LA_Line_C1>"
  Bus Selector/3 -> Bus Creator1/3  "<LA_Line_C2>"
  Bus Selector/4 -> Bus Creator1/4  "<LA_Line_C3>"
  Bus Selector/5 -> Data Type Conversion/1  "<LA_Line_Role>"
  Bus Selector/6 -> Data Type Conversion1/1  "<LA_Lane_Track_ID>"
  Bus Selector/7 -> Data Type Conversion2/1  "<LA_Age>"
  Bus Selector/8 -> Data Type Conversion3/1  "<LA_Color>"
  Bus Selector/9 -> Data Type Conversion4/1  "<LA_Color_Conf>"
  Bus Selector/10 -> Bus Creator1/10  "<LA_Marker_Width>"
  Bus Selector/11 -> Bus Creator1/11  "<LA_Marker_Width_STD>"
  Bus Selector/12 -> Bus Creator1/12  "<LA_View_Range_Start>"
  Bus Selector/13 -> Bus Creator1/13  "<LA_View_Range_End>"
  Bus Selector/14 -> Bus Creator1/14  "<LA_Exist_Probability>"
  Bus Selector/15 -> Data Type Conversion5/1  "<LA_Lanemark_Type>"
  Bus Selector/16 -> Data Type Conversion6/1  "<LA_Lanemark_Type_Conf>"
  Data Type Conversion/1 -> Bus Creator1/5  "LA_Line_Role"
  Data Type Conversion1/1 -> Bus Creator1/6  "LA_Lane_Track_ID"
  Data Type Conversion2/1 -> Bus Creator1/7  "LA_Age"
  Data Type Conversion3/1 -> Bus Creator1/8  "LA_Color"
  Data Type Conversion4/1 -> Bus Creator1/9  "LA_Color_Conf"
  Data Type Conversion5/1 -> Bus Creator1/15  "LA_LaneMark_Type"
  Data Type Conversion6/1 -> Bus Creator1/16  "LA_LaneMark_Type_Conf"
  Bus Selector/17 -> Data Type Conversion7/1  "<LA_DLM_Type>"
  Data Type Conversion7/1 -> Bus Creator1/17  "LA_Type"
